simulink library "lib_HVManager_PostIMG_2017a"  (R2017a)
settings: Solver=VariableStepAuto  StartTime=0.0  StopTime=10.0  RelTol=1e-3
libraries: simulink x12, powerlib_meascontrol x3
settings Model: Creator=Vraj M  LastModifiedBy=vraj

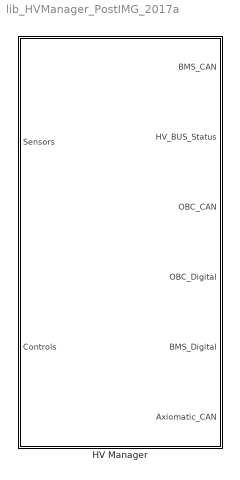
== system lib_HVManager_PostIMG_2017a ==
  HV Manager : Subsystem

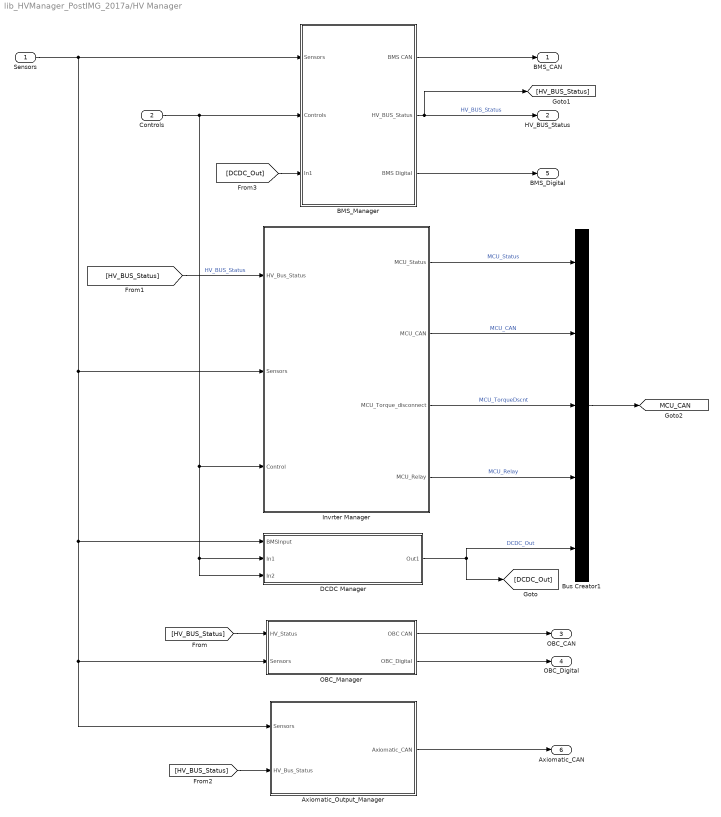
== system lib_HVManager_PostIMG_2017a/HV Manager ==
  Sensors : Inport
  Controls : Inport  Port=2
  Axiomatic_Output_Manager : Subsystem
  BMS_Manager : Subsystem
  Bus Creator1 : BusCreator  Inputs=5
  DCDC Manager : Subsystem
  Invrter Manager : Subsystem
  OBC_Manager : Subsystem
  BMS_CAN : Outport
  HV_BUS_Status : Outport  Port=2
  OBC_CAN : Outport  Port=3
  OBC_Digital : Outport  Port=4
  BMS_Digital : Outport  Port=5
  Axiomatic_CAN : Outport  Port=6
  tag scope: MCU_CAN=global
  wires:
  Axiomatic_Output_Manager/1(Axiomatic_CAN) -> Axiomatic_CAN/1
  BMS_Manager/3(BMS Digital) -> BMS_Digital/1
  BMS_Manager/1(BMS CAN) -> BMS_CAN/1
  Controls/1 -> Invrter Manager/3(Control), DCDC Manager/3(In2), DCDC Manager/2(In1), BMS_Manager/2(Controls)
  OBC_Manager/2(OBC_Digital) -> OBC_Digital/1
  OBC_Manager/1(OBC CAN) -> OBC_CAN/1
  [HV_BUS_Status] -> OBC_Manager/1(HV_Status)
  BMS_Manager/2(HV_BUS_Status) -> HV_BUS_Status/1, [HV_BUS_Status]  "HV_BUS_Status"
  [HV_BUS_Status] -> Axiomatic_Output_Manager/2(HV_Bus_Status)
  [HV_BUS_Status] -> Invrter Manager/1(HV_Bus_Status)  "HV_BUS_Status"
  Sensors/1 -> OBC_Manager/2(Sensors), Axiomatic_Output_Manager/1(Sensors), DCDC Manager/1(BMSInput), Invrter Manager/2(Sensors), BMS_Manager/1(Sensors)
  Invrter Manager/1(MCU_Status) -> Bus Creator1/1  "MCU_Status"
  Invrter Manager/2(MCU_CAN) -> Bus Creator1/2  "MCU_CAN"
  Invrter Manager/3(MCU_Torque_disconnect) -> Bus Creator1/3  "MCU_TorqueDscnt"
  Invrter Manager/4(MCU_Relay) -> Bus Creator1/4  "MCU_Relay"
  Bus Creator1/1 -> [MCU_CAN]
  DCDC Manager/1(Out1) -> Bus Creator1/5, [DCDC_Out]  "DCDC_Out"
  [DCDC_Out] -> BMS_Manager/3(In1)

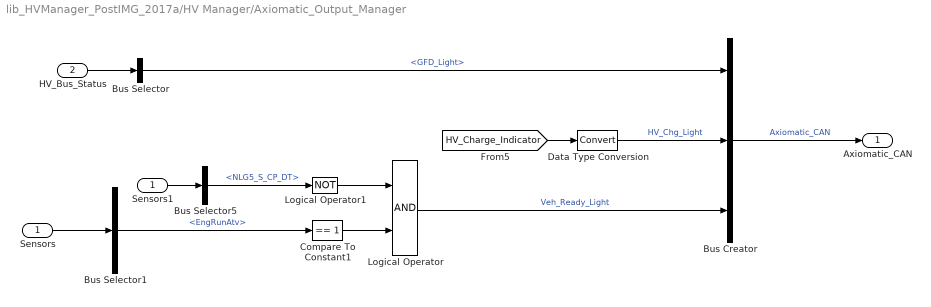
== system lib_HVManager_PostIMG_2017a/HV Manager/Axiomatic_Output_Manager ==
  Sensors : Inport
  HV_Bus_Status : Inport  Port=2
  Bus Creator : BusCreator  Inputs=3
  Bus Selector : BusSelector  OutputSignals=GFD_Light
  Bus Selector1 : BusSelector  OutputSignals=from_CAN.fromEBCAN.from_ECM.EngRunAtv
  Bus Selector5 : BusSelector  OutputSignals=from_CAN.fromHV_CAN.from_OBC.NLG5_ST.NLG5_S_CP_DT
  Compare To Constant1 : simulink/Logic and Bit Operations/Compare To Constant  relop===  const=1  OutDataTypeStr=boolean
      link override Compare: Operator===  OutDataTypeStr=boolean
  Data Type Conversion : DataTypeConversion
  Logical Operator : Logic  AllPortsSameDT=off  OutDataTypeStr=boolean
  Logical Operator1 : Logic  Operator=NOT  AllPortsSameDT=off  OutDataTypeStr=boolean
  Sensors1 : InportShadow
  Axiomatic_CAN : Outport
  wires:
  [HV_Charge_Indicator] -> Data Type Conversion/1
  Sensors/1 -> Bus Selector1/1
  Logical Operator/1 -> Bus Creator/3  "Veh_Ready_Light"
  Data Type Conversion/1 -> Bus Creator/2  "HV_Chg_Light"
  Bus Selector/1 -> Bus Creator/1  "<GFD_Light>"
  Bus Creator/1 -> Axiomatic_CAN/1  "Axiomatic_CAN"
  HV_Bus_Status/1 -> Bus Selector/1
  Compare To Constant1/1 -> Logical Operator/2
  Logical Operator1/1 -> Logical Operator/1
  Bus Selector5/1 -> Logical Operator1/1  "<NLG5_S_CP_DT>"
  Bus Selector1/1 -> Compare To Constant1/1  "<EngRunAtv>"
  Sensors1/1 -> Bus Selector5/1

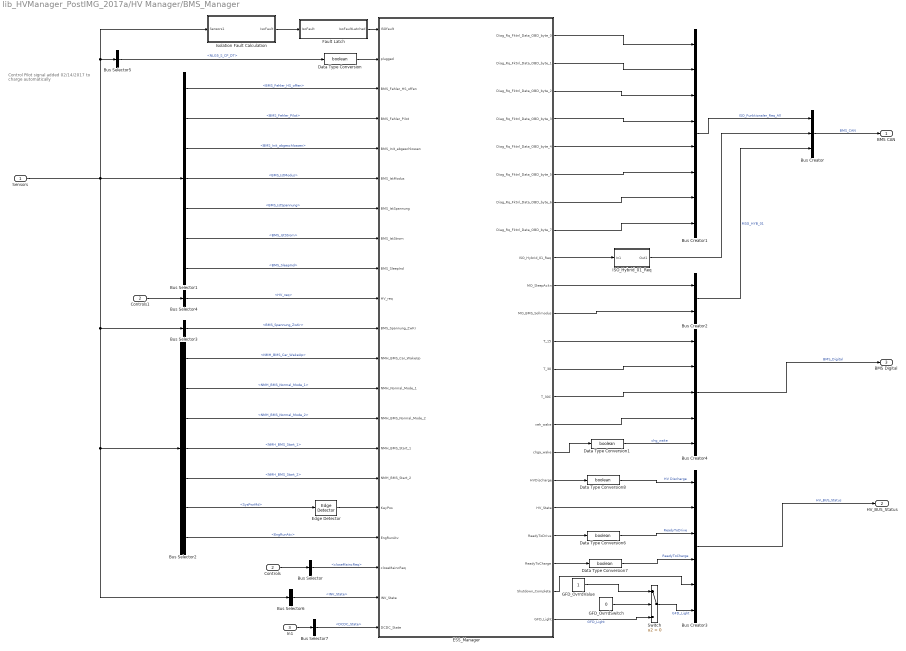
== system lib_HVManager_PostIMG_2017a/HV Manager/BMS_Manager ==
  note: Control Pilot signal added 02/14/2017
      | to charge automatically
  Sensors : Inport
  Controls : Inport  Port=2
  In1 : Inport  Port=3
  Bus Creator : BusCreator  Inputs=3
  Bus Creator1 : BusCreator  Inputs=8
  Bus Creator2 : BusCreator  Inputs=2
  Bus Creator3 : BusCreator  Inputs=6
  Bus Creator4 : BusCreator  Inputs=5
  Bus Selector : BusSelector  OutputSignals=closeMaincReq
  Bus Selector1 : BusSelector  OutputSignals=from_CAN.fromHV_CAN.from_BMSHybrid.BMS_HYB_02.BMS_Fehler_HS_offen,from_CAN.fromHV_CAN.from_BMSHybrid.BMS_HYB_02.BMS_Fehler_Pilot,from_CAN.fromHV_CAN.from_BMSHybrid.BMS_HYB_02.BMS_Init_abgeschlossen,from_CAN.fromHV_CAN.from_BMSHybrid.BMS_HYB_02.BMS_IstModus,from_CAN.fromHV_CAN.from_BMSHybrid.BMS_HYB_02.BMS_IstSpannung,from_CAN.fromHV_CAN.from_BMSHybrid.BMS_HYB_02.BMS_IstStrom,from_CAN.fromHV_CAN.from_BMSHybrid.BMS_HYB_02.BMS_SleepInd
  Bus Selector2 : BusSelector  OutputSignals=from_CAN.fromEBCAN.from_BMSAntrieb.NMH_BMS.NMH_BMS_Car_WakeUp,from_CAN.fromEBCAN.from_BMSAntrieb.NMH_BMS.NMH_BMS_Normal_Mode_1,from_CAN.fromEBCAN.from_BMSAntrieb.NMH_BMS.NMH_BMS_Normal_Mode_2,from_CAN.fromEBCAN.from_BMSAntrieb.NMH_BMS.NMH_BMS_Start_1,from_CAN.fromEBCAN.from_BMSAntrieb.NMH_BMS.NMH_BMS_Start_2,from_CAN.fromVEH_CAN.from_BCM.SysPwrMd,from_CAN.fromEBCAN.from_ECM.EngRunAtv
  Bus Selector3 : BusSelector  OutputSignals=from_CAN.fromHV_CAN.from_BMSHybrid.BMS_Spannung_ZwKr
  Bus Selector4 : BusSelector  OutputSignals=HV_req
  Bus Selector5 : BusSelector  OutputSignals=from_CAN.fromHV_CAN.from_OBC.NLG5_ST.NLG5_S_CP_DT
  Bus Selector6 : BusSelector  OutputSignals=from_CAN.fromHV_CAN.from_MCU.INV_VCU_01.INV_State
  Bus Selector7 : BusSelector  OutputSignals=DCDC_State
  Controls1 : InportShadow  Port=2
  Data Type Conversion{,1,6..8} (5 alike) : DataTypeConversion  OutDataTypeStr=boolean
  ESS_Manager : Stateflow chart  TreatAsAtomicUnit=on
  Edge Detector : powerlib_meascontrol/Logic/Edge Detector  model=Either  ic=0  Ts=0
      settings: SourceProductName=Simscape Power Systems  SourceProductBaseCode=PS
  Fault Latch : Subsystem
  GFD_OvrrdSwitch : Constant  Value=0
  GFD_OvrrdValue : Constant
  ISO_Hybrid_01_Req : Subsystem
  Isolation Fault Calculation : Subsystem
  Switch : Switch  Criteria=u2 > Threshold
  BMS CAN : Outport
  HV_BUS_Status : Outport  Port=2
  BMS Digital : Outport  Port=3
  wires:
  ISO_Hybrid_01_Req/1(Out1) -> Bus Creator/2
  ESS_Manager/9(ISO_Hybrid_01_Req) -> ISO_Hybrid_01_Req/1(In1)
  ESS_Manager/11(MO_BMS_Sollmodus) -> Bus Creator2/2
  Sensors/1 -> Bus Selector6/1, Bus Selector2/1, Bus Selector3/1, Isolation Fault Calculation/1(Sensors1), Bus Selector5/1, Bus Selector1/1
  Data Type Conversion1/1 -> Bus Creator4/5  "chg_wake"
  Bus Creator4/1 -> BMS Digital/1  "BMS_Digital"
  Bus Creator/1 -> BMS CAN/1  "BMS_CAN"
  Controls1/1 -> Bus Selector4/1
  Bus Selector/1 -> ESS_Manager/19(closeMaincReq)  "<closeMaincReq>"
  Controls/1 -> Bus Selector/1
  Bus Creator3/1 -> HV_BUS_Status/1  "HV_BUS_Status"
  ESS_Manager/18(HV_State) -> Bus Creator3/2
  ESS_Manager/15(veh_wake) -> Bus Creator4/4
  ESS_Manager/14(T_30C) -> Bus Creator4/3
  ESS_Manager/16(chga_wake) -> Data Type Conversion1/1
  ESS_Manager/13(T_30) -> Bus Creator4/2
  ESS_Manager/21(Shutdown_Complete) -> Bus Creator3/5
  ESS_Manager/20(ReadyToCharge) -> Data Type Conversion7/1
  ESS_Manager/19(ReadyToDrive) -> Data Type Conversion6/1
  ESS_Manager/17(HVDischarge) -> Data Type Conversion8/1
  Bus Creator1/1 -> Bus Creator/1  "ISO_Funktionaler_Req_All"
  Data Type Conversion8/1 -> Bus Creator3/1  "HV Discharge"
  Data Type Conversion7/1 -> Bus Creator3/4  "ReadyToCharge"
  Data Type Conversion6/1 -> Bus Creator3/3  "ReadyToDrive"
  ESS_Manager/12(T_15) -> Bus Creator4/1
  ESS_Manager/10(MO_SleepAckn) -> Bus Creator2/1
  ESS_Manager/8(Diag_Rq_Fktnl_Data_OBD_byte_7) -> Bus Creator1/8
  ESS_Manager/7(Diag_Rq_Fktnl_Data_OBD_byte_6) -> Bus Creator1/7
  ESS_Manager/6(Diag_Rq_Fktnl_Data_OBD_byte_5) -> Bus Creator1/6
  ESS_Manager/5(Diag_Rq_Fktnl_Data_OBD_byte_4) -> Bus Creator1/5
  ESS_Manager/4(Diag_Rq_Fktnl_Data_OBD_byte_3) -> Bus Creator1/4
  ESS_Manager/3(Diag_Rq_Fktnl_Data_OBD_byte_2) -> Bus Creator1/3
  ESS_Manager/2(Diag_Rq_Fktnl_Data_OBD_byte_1) -> Bus Creator1/2
  ESS_Manager/1(Diag_Rq_Fktnl_Data_OBD_byte_0) -> Bus Creator1/1
  Bus Selector5/1 -> Data Type Conversion/1  "<NLG5_S_CP_DT>"
  Bus Selector3/1 -> ESS_Manager/11(BMS_Spannung_ZwKr)  "<BMS_Spannung_ZwKr>"
  Bus Selector2/3 -> ESS_Manager/14(NMH_BMS_Normal_Mode_2)  "<NMH_BMS_Normal_Mode_2>"
  Bus Selector2/2 -> ESS_Manager/13(NMH_Normal_Mode_1)  "<NMH_BMS_Normal_Mode_1>"
  Bus Selector2/1 -> ESS_Manager/12(NMH_BMS_Car_WakeUp)  "<NMH_BMS_Car_WakeUp>"
  Bus Selector1/5 -> ESS_Manager/7(BMS_IstSpannung)  "<BMS_IstSpannung>"
  Bus Selector1/4 -> ESS_Manager/6(BMS_IstModus)  "<BMS_IstModus>"
  Bus Selector1/3 -> ESS_Manager/5(BMS_Init_abgeschlossen)  "<BMS_Init_abgeschlossen>"
  Bus Selector1/2 -> ESS_Manager/4(BMS_Fehler_Pilot)  "<BMS_Fehler_Pilot>"
  Bus Selector1/1 -> ESS_Manager/3(BMS_Fehler_HS_offen)  "<BMS_Fehler_HS_offen>"
  Switch/1 -> Bus Creator3/6  "GFD_Light"
  Isolation Fault Calculation/1(IsoFault) -> Fault Latch/1(IsoFault)
  Fault Latch/1(IsoFaultLatched) -> ESS_Manager/1(ISOfault)
  Bus Creator2/1 -> Bus Creator/3  "MSG_HYB_01"
  Bus Selector4/1 -> ESS_Manager/10(HV_req)  "<HV_req>"
  Bus Selector2/6 -> Edge Detector/1  "<SysPwrMd>"
  Edge Detector/1 -> ESS_Manager/17(KeyPos)
  Bus Selector2/7 -> ESS_Manager/18(EngRunAtv)  "<EngRunAtv>"
  Bus Selector2/5 -> ESS_Manager/16(NMH_BMS_Start_2)  "<NMH_BMS_Start_2>"
  Bus Selector2/4 -> ESS_Manager/15(NMH_BMS_Start_1)  "<NMH_BMS_Start_1>"
  Bus Selector1/7 -> ESS_Manager/9(BMS_SleepInd)  "<BMS_SleepInd>"
  Bus Selector1/6 -> ESS_Manager/8(BMS_IstStrom)  "<BMS_IstStrom>"
  Data Type Conversion/1 -> ESS_Manager/2(plugged)
  ESS_Manager/22(GFD_Light) -> Switch/3  "GFD_Light"
  GFD_OvrrdSwitch/1 -> Switch/2
  GFD_OvrrdValue/1 -> Switch/1
  Bus Selector6/1 -> ESS_Manager/20(INV_State)  "<INV_State>"
  In1/1 -> Bus Selector7/1
  Bus Selector7/1 -> ESS_Manager/21(DCDC_State)  "<DCDC_State>"

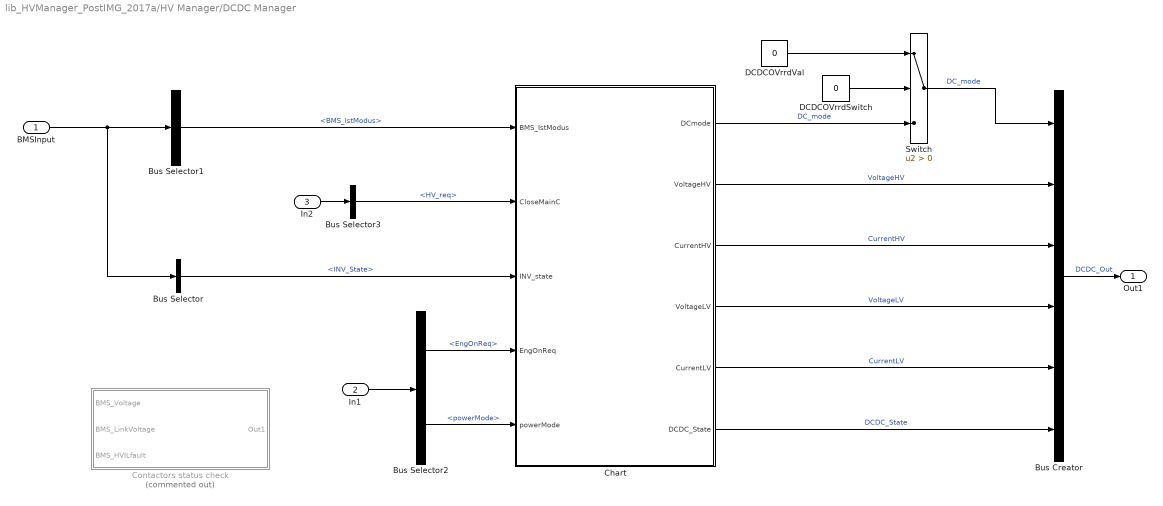
== system lib_HVManager_PostIMG_2017a/HV Manager/DCDC Manager ==
  BMSInput : Inport
  In1 : Inport  Port=2
  In2 : Inport  Port=3
  Bus Creator : BusCreator  Inputs=6
  Bus Selector : BusSelector  OutputSignals=from_CAN.fromHV_CAN.from_MCU.INV_VCU_01.INV_State
  Bus Selector1 : BusSelector  OutputSignals=from_CAN.fromHV_CAN.from_BMSHybrid.BMS_HYB_02.BMS_IstModus
  Bus Selector2 : BusSelector  OutputSignals=EngOnReq,powerMode
  Bus Selector3 : BusSelector  OutputSignals=HV_req
  Chart : Stateflow chart  RequirementInfo={} %GIDa_d26a8659_2f91_4e0f_9a85_a466cd76580c  TreatAsAtomicUnit=on
  Contactors status check : Subsystem  Commented=on
  DCDCOVrrdSwitch : Constant  Value=0
  DCDCOVrrdVal : Constant  Value=0
  Switch : Switch  Criteria=u2 > Threshold
  Out1 : Outport
  wires:
  BMSInput/1 -> Bus Selector/1, Bus Selector1/1
  Bus Selector/1 -> Chart/3(INV_state)  "<INV_State>"
  Switch/1 -> Bus Creator/1  "DC_mode"
  Chart/5(CurrentLV) -> Bus Creator/5  "CurrentLV"
  Chart/4(VoltageLV) -> Bus Creator/4  "VoltageLV"
  Chart/3(CurrentHV) -> Bus Creator/3  "CurrentHV"
  Chart/2(VoltageHV) -> Bus Creator/2  "VoltageHV"
  Bus Creator/1 -> Out1/1  "DCDC_Out"
  Chart/6(DCDC_State) -> Bus Creator/6  "DCDC_State"
  Chart/1(DCmode) -> Switch/3  "DC_mode"
  DCDCOVrrdSwitch/1 -> Switch/2
  DCDCOVrrdVal/1 -> Switch/1
  In1/1 -> Bus Selector2/1
  Bus Selector2/2 -> Chart/5(powerMode)  "<powerMode>"
  Bus Selector1/1 -> Chart/1(BMS_IstModus)  "<BMS_IstModus>"
  Bus Selector2/1 -> Chart/4(EngOnReq)  "<EngOnReq>"
  In2/1 -> Bus Selector3/1
  Bus Selector3/1 -> Chart/2(CloseMainC)  "<HV_req>"

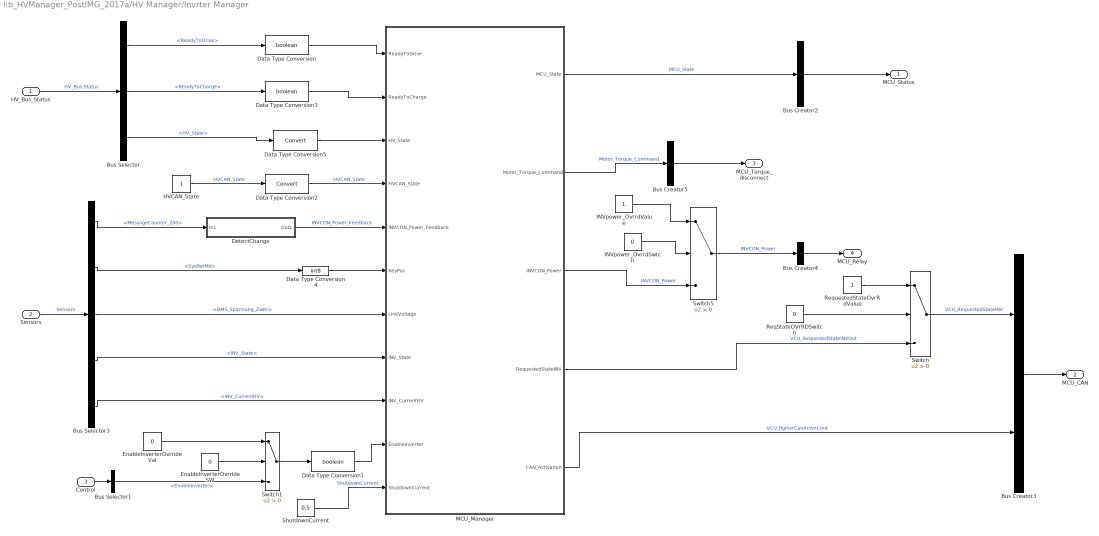
== system lib_HVManager_PostIMG_2017a/HV Manager/Invrter Manager ==
  HV_Bus_Status : Inport
  Sensors : Inport  Port=2
  Control : Inport  Port=3
  Bus Creator2 : BusCreator  Inputs=1
  Bus Creator3 : BusCreator  Inputs=2
  Bus Creator4 : BusCreator  Inputs=1
  Bus Creator5 : BusCreator  Inputs=1
  Bus Selector : BusSelector  OutputSignals=ReadyToDrive,ReadyToCharge,HV_State
  Bus Selector1 : BusSelector  OutputSignals=EnableInverter
  Bus Selector3 : BusSelector  OutputSignals=from_CAN.fromHV_CAN.from_MCU.INV_VCU_01.MessageCounter_200,from_CAN.fromVEH_CAN.from_BCM.SysPwrMd,from_CAN.fromHV_CAN.from_BMSHybrid.BMS_Spannung_ZwKr,from_CAN.fromHV_CAN.from_MCU.INV_VCU_01.INV_State,from_CAN.fromHV_CAN.from_MCU.INV_VCU_01.INV_CurrentHV
  Data Type Conversion : DataTypeConversion  OutDataTypeStr=boolean
  Data Type Conversion1 : DataTypeConversion  OutDataTypeStr=boolean
  Data Type Conversion2 : DataTypeConversion
  Data Type Conversion3 : DataTypeConversion  OutDataTypeStr=boolean
  Data Type Conversion4 : DataTypeConversion  OutDataTypeStr=int8
  Data Type Conversion5 : DataTypeConversion
  DetectChange : Subsystem
  EnableInverterOvrrideSW : Constant  Value=0
  EnableInverterOvrrideVal : Constant  Value=0
  HVCAN_State : Constant
  INVpower_OvrrdSwtch : Constant  Value=0
  INVpower_OvrrdValue : Constant
  "MCU_Manager " : Stateflow chart  RequirementInfo={} %GIDa_847f7ea3_a24c_4f3c_837a_ca9eed8e7071  TreatAsAtomicUnit=on
  ReqStateOVrRDSwitch : Constant  Value=0
  RequestedStateOvrRdValue : Constant
  ShutdownCurrent : Constant  Value=0.5
  Switch : Switch  Criteria=u2 > Threshold
  Switch1 : Switch  Criteria=u2 > Threshold
  Switch5 : Switch  Criteria=u2 > Threshold
  MCU_Status : Outport
  MCU_CAN : Outport  Port=2
  MCU_Torque_disconnect : Outport  Port=3
  MCU_Relay : Outport  Port=4
  wires:
  HVCAN_State/1 -> Data Type Conversion2/1  "HVCAN_State"
  Bus Selector3/4 -> "MCU_Manager "/8(INV_State)  "<INV_State>"
  Data Type Conversion1/1 -> "MCU_Manager "/10(EnableInverter)
  Data Type Conversion/1 -> "MCU_Manager "/1(ReadyToDrive)
  Bus Creator5/1 -> MCU_Torque_disconnect/1
  "MCU_Manager "/2(Motor_Torque_Command) -> Bus Creator5/1  "Motor_Torque_Command"
  Bus Creator4/1 -> MCU_Relay/1
  Switch5/1 -> Bus Creator4/1  "INVCON_Power"
  Bus Creator2/1 -> MCU_Status/1
  "MCU_Manager "/1(MCU_State) -> Bus Creator2/1  "MCU_State"
  Bus Selector3/5 -> "MCU_Manager "/9(INV_CurrentHV)  "<INV_CurrentHV>"
  ShutdownCurrent/1 -> "MCU_Manager "/11(ShutdownCurrent)  "ShutdownCurrent"
  Bus Selector/1 -> Data Type Conversion/1  "<ReadyToDrive>"
  HV_Bus_Status/1 -> Bus Selector/1  "HV_Bus Status"
  EnableInverterOvrrideVal/1 -> Switch1/1
  Sensors/1 -> Bus Selector3/1  "Sensors"
  Bus Creator3/1 -> MCU_CAN/1
  Data Type Conversion2/1 -> "MCU_Manager "/4(HVCAN_State)  "HVCAN_State"
  Bus Selector/2 -> Data Type Conversion3/1  "<ReadyToCharge>"
  Data Type Conversion3/1 -> "MCU_Manager "/2(ReadyToCharge)
  DetectChange/1(Out1) -> "MCU_Manager "/5(INVCON_Power_Feedback)  "INVCON_Power_Feedback"
  "MCU_Manager "/5(CAN_Activation) -> Bus Creator3/2  "VCU_flgInvrCanActvnCmd"
  Switch/1 -> Bus Creator3/1  "VCU_RequestedStateINV"
  "MCU_Manager "/4(RequestedStateINV) -> Switch/3  "VCU_RequestedStateINVOut"
  ReqStateOVrRDSwitch/1 -> Switch/2
  RequestedStateOvrRdValue/1 -> Switch/1
  Control/1 -> Bus Selector1/1
  Switch1/1 -> Data Type Conversion1/1
  Bus Selector1/1 -> Switch1/3  "<EnableInverter>"
  EnableInverterOvrrideSW/1 -> Switch1/2
  Bus Selector3/3 -> "MCU_Manager "/7(LinkVoltage)  "<BMS_Spannung_ZwKr>"
  Bus Selector3/2 -> Data Type Conversion4/1  "<SysPwrMd>"
  Data Type Conversion4/1 -> "MCU_Manager "/6(KeyPos)
  Bus Selector3/1 -> DetectChange/1(In1)  "<MessageCounter_200>"
  Bus Selector/3 -> Data Type Conversion5/1  "<HV_State>"
  Data Type Conversion5/1 -> "MCU_Manager "/3(HV_State)
  INVpower_OvrrdSwtch/1 -> Switch5/2
  INVpower_OvrrdValue/1 -> Switch5/1
  "MCU_Manager "/3(INVCON_Power) -> Switch5/3  "INVCON_Power"

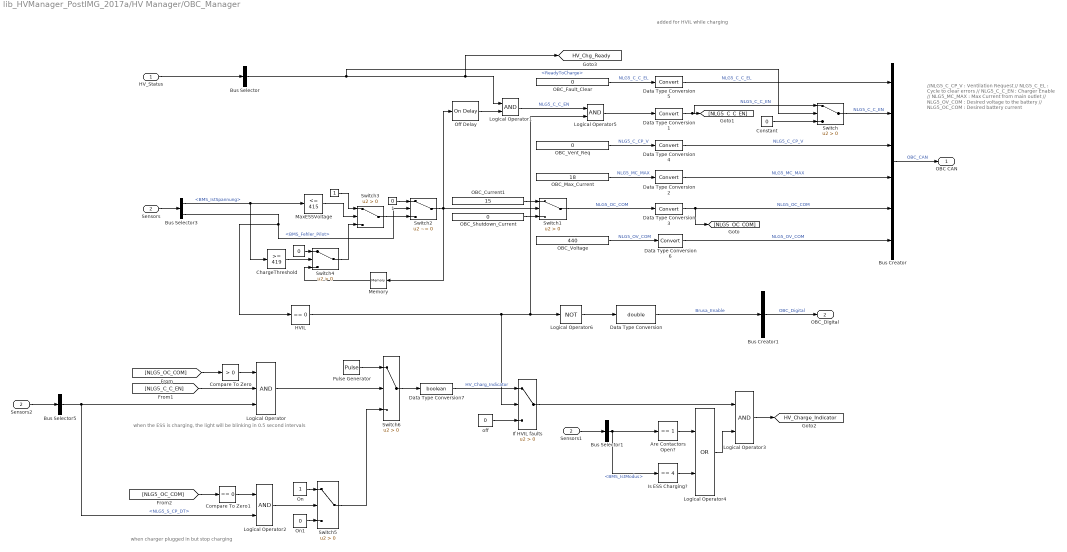
== system lib_HVManager_PostIMG_2017a/HV Manager/OBC_Manager ==
  note: added for HVIL
      | while charging
  note: //NLG5_C_CP_V : Ventilation Request
      | // NLG5_C_EL : Cycle to clear errors
      | // NLG5_C_C_EN : Charger Enable
      | // NLG5_MC_MAX : Max Current from main outlet
      | // NLG5_OV_COM : Desired voltage to the battery
      | // NLG5_OC_COM : Desired battery current
  note: when charger plugged in but stop charging
  note: when the ESS is charging, the light will be blinking in 0.5 second intervals
  HV_Status : Inport
  Sensors : Inport  Port=2
  " " : Constant
  "   " : Constant  Value=0
  "   1" : Constant  Value=0
  Are Contactors Open? : simulink/Logic and Bit Operations/Compare To Constant  relop===  const=1  OutDataTypeStr=boolean
      link override Compare: Operator===  OutDataTypeStr=boolean
  Bus Creator : BusCreator  Inputs=6
  Bus Creator1 : BusCreator  Inputs=1
  Bus Selector : BusSelector  OutputSignals=ReadyToCharge
  Bus Selector1 : BusSelector  OutputSignals=from_CAN.fromHV_CAN.from_BMSHybrid.BMS_HYB_02.BMS_IstModus
  Bus Selector3 : BusSelector  OutputSignals=from_CAN.fromHV_CAN.from_BMSHybrid.BMS_HYB_02.BMS_IstSpannung,from_CAN.fromHV_CAN.from_BMSHybrid.BMS_HYB_02.BMS_Fehler_Pilot
  Bus Selector5 : BusSelector  OutputSignals=from_CAN.fromHV_CAN.from_OBC.NLG5_ST.NLG5_S_CP_DT
  ChargeThreshold : simulink/Logic and Bit Operations/Compare To Constant  relop=>=  const=419  OutDataTypeStr=boolean
      link override Compare: Operator=>=  OutDataTypeStr=boolean
  Compare To Zero : simulink/Logic and Bit Operations/Compare To Zero  relop=>  OutDataTypeStr=boolean
      link override Compare: Operator=>  OutDataTypeStr=boolean
  Compare To Zero1 : simulink/Logic and Bit Operations/Compare To Zero  relop===  OutDataTypeStr=boolean
      link override Compare: Operator===  OutDataTypeStr=boolean
  Constant : Constant  Value=0
  Data Type Conversion : DataTypeConversion  OutDataTypeStr=double
  Data Type Conversion{1..6} (6 alike) : DataTypeConversion
  Data Type Conversion7 : DataTypeConversion  OutDataTypeStr=boolean
  HVIL : simulink/Logic and Bit Operations/Compare To Constant  relop===  const=0  OutDataTypeStr=boolean
      link override Compare: Operator===  OutDataTypeStr=boolean
  If HVIL faults : Switch  Criteria=u2 > Threshold
  Is ESS Charging? : simulink/Logic and Bit Operations/Compare To Constant  relop===  const=4  OutDataTypeStr=boolean
      link override Compare: Operator===  OutDataTypeStr=boolean
  Logical Operator : Logic  Inputs=3  AllPortsSameDT=off  OutDataTypeStr=boolean
  Logical Operator{1..3,5} (4 alike) : Logic  AllPortsSameDT=off  OutDataTypeStr=boolean
  Logical Operator4 : Logic  Operator=OR  AllPortsSameDT=off  OutDataTypeStr=boolean
  Logical Operator6 : Logic  Operator=NOT  Inputs=3  AllPortsSameDT=off  OutDataTypeStr=boolean
  MaxESSVoltage : simulink/Logic and Bit Operations/Compare To Constant  relop=<=  const=415  OutDataTypeStr=boolean
      link override Compare: Operator=<=  OutDataTypeStr=boolean
  Memory : Memory  InheritSampleTime=on
  OBC_Current1 : Constant  Value=15
  OBC_Fault_Clear : Constant  Value=0
  OBC_Max_Current : Constant  Value=18
  OBC_Shutdown_Current : Constant  Value=0
  OBC_Vent_Req : Constant  Value=0
  OBC_Voltage : Constant  Value=440
  Off Delay : powerlib_meascontrol/Logic/On Delay  DelayType=Off delay  delay=30  ic=0  Ts=0
      settings: SourceProductName=Simscape Power Systems
  On : Constant
  On1 : Constant  Value=0
  Pulse Generator : DiscretePulseGenerator  PulseType=Time based  Period=1  PulseWidth=50
  Sensors1 : InportShadow  Port=2
  Sensors2 : InportShadow  Port=2
  Switch{,1,3..6} (6 alike) : Switch  Criteria=u2 > Threshold
  Switch2 : Switch  Criteria=u2 ~= 0
  off : Constant  Value=0
  OBC CAN : Outport
  OBC_Digital : Outport  Port=2
  tag scope: HV_Charge_Indicator=global, HV_Chg_Ready=global
  wires:
  Data Type Conversion7/1 -> If HVIL faults/1  "HV_Charg_Indicator"
  OBC_Voltage/1 -> Data Type Conversion6/1  "NLG5_OV_COM"
  OBC_Max_Current/1 -> Data Type Conversion2/1  "NLG5_MC_MAX"
  OBC_Fault_Clear/1 -> Data Type Conversion5/1  "NLG5_C_C_EL"
  OBC_Vent_Req/1 -> Data Type Conversion4/1  "NLG5_C_CP_V"
  Switch1/1 -> Data Type Conversion3/1  "NLG5_OC_COM"
  Logical Operator1/1 -> Logical Operator5/1  "NLG5_C_C_EN"
  Data Type Conversion1/1 -> Switch/1, [NLG5_C_C_EN]  "NLG5_C_C_EN"
  Switch4/1 -> Switch3/3
  Memory/1 -> Switch4/3
  OBC_Shutdown_Current/1 -> Switch1/3
  " "/1 -> Switch3/1
  ChargeThreshold/1 -> Switch4/2
  "   "/1 -> Switch4/1
  Switch2/1 -> Memory/1, Off Delay/1, Switch1/2
  OBC_Current1/1 -> Switch1/1
  Data Type Conversion3/1 -> Bus Creator/5, [NLG5_OC_COM]  "NLG5_OC_COM"
  Data Type Conversion6/1 -> Bus Creator/6  "NLG5_OV_COM"
  Data Type Conversion4/1 -> Bus Creator/3  "NLG5_C_CP_V"
  Data Type Conversion5/1 -> Bus Creator/1  "NLG5_C_C_EL"
  Data Type Conversion2/1 -> Bus Creator/4  "NLG5_MC_MAX"
  Bus Selector3/1 -> ChargeThreshold/1, MaxESSVoltage/1  "<BMS_IstSpannung>"
  Off Delay/1 -> Logical Operator1/2
  Bus Selector/1 -> Switch/2, Logical Operator1/1, [HV_Chg_Ready]  "<ReadyToCharge>"
  MaxESSVoltage/1 -> Switch3/2
  HV_Status/1 -> Bus Selector/1
  Bus Creator/1 -> OBC CAN/1  "OBC_CAN"
  Sensors/1 -> Bus Selector3/1
  [NLG5_OC_COM] -> Compare To Zero/1
  Compare To Zero/1 -> Logical Operator/1
  [NLG5_C_C_EN] -> Logical Operator/2
  Logical Operator/1 -> Switch6/2
  Pulse Generator/1 -> Switch6/1
  [NLG5_OC_COM] -> Compare To Zero1/1
  Compare To Zero1/1 -> Logical Operator2/1
  Logical Operator2/1 -> Switch5/2
  On/1 -> Switch5/1
  On1/1 -> Switch5/3
  Switch5/1 -> Switch6/3
  Switch6/1 -> Data Type Conversion7/1
  Bus Selector3/2 -> HVIL/1, Switch2/2  "<BMS_Fehler_Pilot>"
  Data Type Conversion/1 -> Bus Creator1/1  "Brusa_Enable"
  Bus Creator1/1 -> OBC_Digital/1  "OBC_Digital"
  Switch3/1 -> Switch2/3
  "   1"/1 -> Switch2/1
  HVIL/1 -> Logical Operator5/2, Logical Operator6/1, If HVIL faults/2
  If HVIL faults/1 -> Logical Operator3/1
  off/1 -> If HVIL faults/3
  Logical Operator3/1 -> [HV_Charge_Indicator]
  Sensors1/1 -> Bus Selector1/1
  Are Contactors Open?/1 -> Logical Operator4/1
  Bus Selector1/1 -> Is ESS Charging?/1, Are Contactors Open?/1  "<BMS_IstModus>"
  Is ESS Charging?/1 -> Logical Operator4/2
  Logical Operator4/1 -> Logical Operator3/2
  Logical Operator5/1 -> Data Type Conversion1/1
  Logical Operator6/1 -> Data Type Conversion/1
  Constant/1 -> Switch/3
  Switch/1 -> Bus Creator/2  "NLG5_C_C_EN"
  Bus Selector5/1 -> Logical Operator2/2, Logical Operator/3  "<NLG5_S_CP_DT>"
  Sensors2/1 -> Bus Selector5/1

== system lib_HVManager_PostIMG_2017a/HV Manager/BMS_Manager/Fault Latch ==
  IsoFault : Inport
  Off Delay : powerlib_meascontrol/Logic/On Delay  DelayType=Off delay  delay=3  ic=0  Ts=0
      settings: SourceProductName=Simscape Power Systems
  IsoFaultLatched : Outport
  wires:
  IsoFault/1 -> Off Delay/1
  Off Delay/1 -> IsoFaultLatched/1

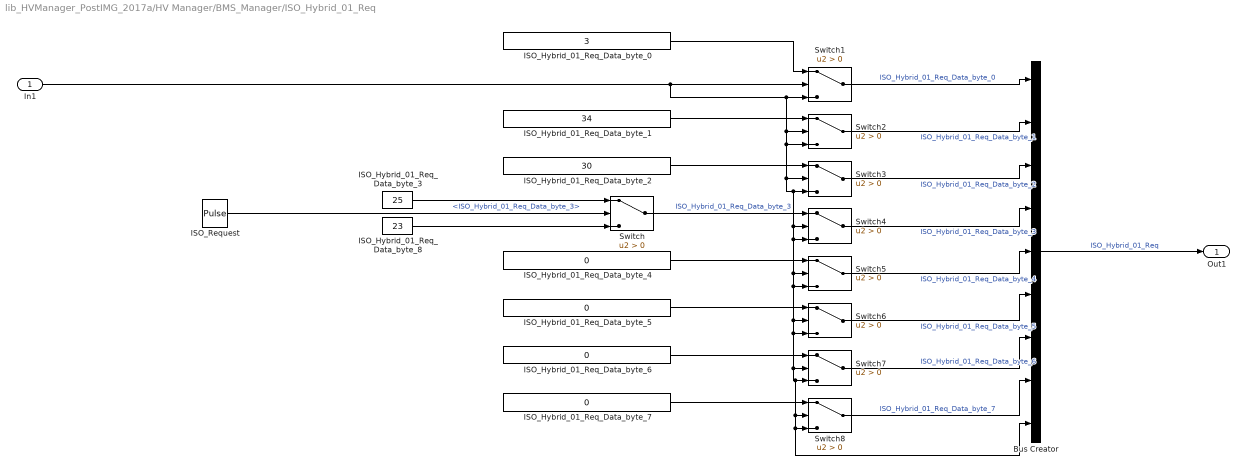
== system lib_HVManager_PostIMG_2017a/HV Manager/BMS_Manager/ISO_Hybrid_01_Req ==
  In1 : Inport
  Bus Creator : BusCreator  Inputs=9
  ISO_Hybrid_01_Req_Data_byte_0 : Constant  Value=3
  ISO_Hybrid_01_Req_Data_byte_1 : Constant  Value=34
  ISO_Hybrid_01_Req_Data_byte_2 : Constant  Value=30
  ISO_Hybrid_01_Req_Data_byte_3 : Constant  Value=25
  ISO_Hybrid_01_Req_Data_byte_{4..7} (4 alike) : Constant  Value=0
  ISO_Hybrid_01_Req_Data_byte_8 : Constant  Value=23
  ISO_Request : DiscretePulseGenerator  PulseType=Time based  Period=0.5  PulseWidth=50  SampleTime=-1
  Switch{,1..8} (9 alike) : Switch  Criteria=u2 > Threshold
  Out1 : Outport
  wires:
  Bus Creator/1 -> Out1/1  "ISO_Hybrid_01_Req"
  Switch6/1 -> Bus Creator/6  "ISO_Hybrid_01_Req_Data_byte_5"
  ISO_Hybrid_01_Req_Data_byte_8/1 -> Switch/3
  Switch5/1 -> Bus Creator/5  "ISO_Hybrid_01_Req_Data_byte_4"
  Switch3/1 -> Bus Creator/3  "ISO_Hybrid_01_Req_Data_byte_2"
  ISO_Hybrid_01_Req_Data_byte_3/1 -> Switch/1
  Switch1/1 -> Bus Creator/1  "ISO_Hybrid_01_Req_Data_byte_0"
  Switch7/1 -> Bus Creator/7  "ISO_Hybrid_01_Req_Data_byte_6"
  Switch2/1 -> Bus Creator/2  "ISO_Hybrid_01_Req_Data_byte_1"
  Switch8/1 -> Bus Creator/8  "ISO_Hybrid_01_Req_Data_byte_7"
  Switch4/1 -> Bus Creator/4  "ISO_Hybrid_01_Req_Data_byte_3"
  ISO_Hybrid_01_Req_Data_byte_0/1 -> Switch1/1
  In1/1 -> Switch2/2, Switch3/3, Switch4/3, Switch5/3, Switch6/3, Switch7/2, Switch7/3, Switch8/2, Bus Creator/9, Switch8/3, Switch6/2, Switch5/2, Switch4/2, Switch3/2, Switch2/3, Switch1/3, Switch1/2
  ISO_Hybrid_01_Req_Data_byte_1/1 -> Switch2/1
  ISO_Hybrid_01_Req_Data_byte_2/1 -> Switch3/1
  Switch/1 -> Switch4/1  "ISO_Hybrid_01_Req_Data_byte_3"
  ISO_Hybrid_01_Req_Data_byte_4/1 -> Switch5/1
  ISO_Hybrid_01_Req_Data_byte_5/1 -> Switch6/1
  ISO_Hybrid_01_Req_Data_byte_6/1 -> Switch7/1
  ISO_Hybrid_01_Req_Data_byte_7/1 -> Switch8/1
  ISO_Request/1 -> Switch/2  "<ISO_Hybrid_01_Req_Data_byte_3>"

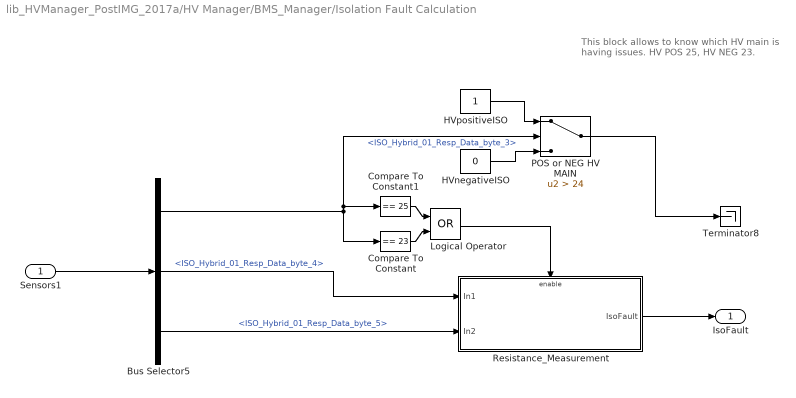
== system lib_HVManager_PostIMG_2017a/HV Manager/BMS_Manager/Isolation Fault Calculation ==
  note: This block  allows to know which HV main
      | is having issues. HV POS 25, HV NEG 23.
  Sensors1 : Inport
  Bus Selector5 : BusSelector  OutputSignals=from_CAN.fromEBCAN.from_BMSAntrieb.ISO_Hybrid_01_Resp_Data.ISO_Hybrid_01_Resp_Data_byte_3,from_CAN.fromEBCAN.from_BMSAntrieb.ISO_Hybrid_01_Resp_Data.ISO_Hybrid_01_Resp_Data_byte_4,from_CAN.fromEBCAN.from_BMSAntrieb.ISO_Hybrid_01_Resp_Data.ISO_Hybrid_01_Resp_Data_byte_5
  Compare To Constant : simulink/Logic and Bit Operations/Compare To Constant  relop===  const=23  OutDataTypeStr=boolean
      link override Compare: Operator===  OutDataTypeStr=boolean
  Compare To Constant1 : simulink/Logic and Bit Operations/Compare To Constant  relop===  const=25  OutDataTypeStr=boolean
      link override Compare: Operator===  OutDataTypeStr=boolean
  HVnegativeISO : Constant  Value=0
  HVpositiveISO : Constant
  Logical Operator : Logic  Operator=OR  AllPortsSameDT=off  OutDataTypeStr=boolean
  POS or NEG HV MAIN : Switch  Criteria=u2 > Threshold  Threshold=24
  Resistance_Measurement : Subsystem
  Terminator8 : Terminator
  IsoFault : Outport
  wires:
  Resistance_Measurement/1(IsoFault) -> IsoFault/1
  POS or NEG HV MAIN/1 -> Terminator8/1
  Bus Selector5/2 -> Resistance_Measurement/1(In1)  "<ISO_Hybrid_01_Resp_Data_byte_4>"
  Bus Selector5/3 -> Resistance_Measurement/2(In2)  "<ISO_Hybrid_01_Resp_Data_byte_5>"
  Sensors1/1 -> Bus Selector5/1
  HVpositiveISO/1 -> POS or NEG HV MAIN/1
  Bus Selector5/1 -> POS or NEG HV MAIN/2, Compare To Constant1/1, Compare To Constant/1  "<ISO_Hybrid_01_Resp_Data_byte_3>"
  HVnegativeISO/1 -> POS or NEG HV MAIN/3
  Compare To Constant1/1 -> Logical Operator/1
  Compare To Constant/1 -> Logical Operator/2
  Logical Operator/1 -> Resistance_Measurement/Enable

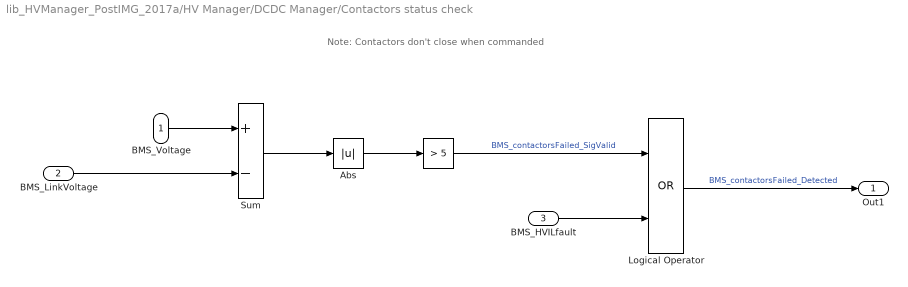
== system lib_HVManager_PostIMG_2017a/HV Manager/DCDC Manager/Contactors status check ==
  note: Note: Contactors don't close when commanded
  BMS_Voltage : Inport
  BMS_LinkVoltage : Inport  Port=2
  BMS_HVILfault : Inport  Port=3
  " " : simulink/Logic and Bit Operations/Compare To Constant  relop=>  const=5  OutDataTypeStr=boolean
      link override Compare: Operator=>  OutDataTypeStr=boolean
  Abs : Abs
  Logical Operator : Logic  Operator=OR  AllPortsSameDT=off  OutDataTypeStr=boolean
  Sum : Sum  Inputs=+-
  Out1 : Outport
  wires:
  BMS_Voltage/1 -> Sum/1
  Logical Operator/1 -> Out1/1  "BMS_contactorsFailed_Detected"
  Sum/1 -> Abs/1
  Abs/1 -> " "/1
  BMS_LinkVoltage/1 -> Sum/2
  BMS_HVILfault/1 -> Logical Operator/2
  " "/1 -> Logical Operator/1  "BMS_contactorsFailed_SigValid"

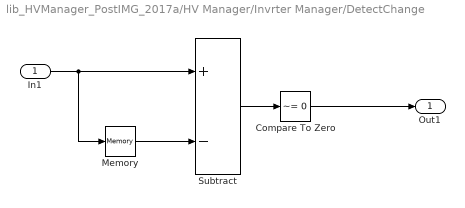
== system lib_HVManager_PostIMG_2017a/HV Manager/Invrter Manager/DetectChange ==
  In1 : Inport
  Compare To Zero : simulink/Logic and Bit Operations/Compare To Zero  relop=~=  OutDataTypeStr=boolean
  Memory : Memory
  Subtract : Sum  Inputs=+-
  Out1 : Outport
  wires:
  Memory/1 -> Subtract/2
  Compare To Zero/1 -> Out1/1
  Subtract/1 -> Compare To Zero/1
  In1/1 -> Subtract/1, Memory/1

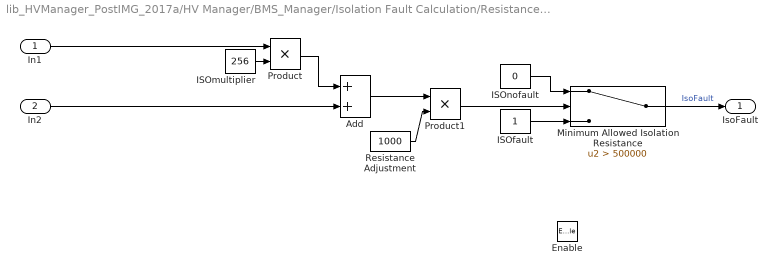
== system lib_HVManager_PostIMG_2017a/HV Manager/BMS_Manager/Isolation Fault Calculation/Resistance_Measurement ==
  In1 : Inport
  In2 : Inport  Port=2
  Enable : EnablePort
  Add : Sum
  ISOfault : Constant
  ISOmultiplier : Constant  Value=256
  ISOnofault : Constant  Value=0
  Minimum Allowed Isolation Resistance : Switch  Criteria=u2 > Threshold  Threshold=500000
  Product : Product
  Product1 : Product
  Resistance Adjustment : Constant  Value=1000
  IsoFault : Outport
  wires:
  Minimum Allowed Isolation Resistance/1 -> IsoFault/1  "IsoFault"
  ISOnofault/1 -> Minimum Allowed Isolation Resistance/1
  Resistance Adjustment/1 -> Product1/2
  Product1/1 -> Minimum Allowed Isolation Resistance/2
  ISOfault/1 -> Minimum Allowed Isolation Resistance/3
  Add/1 -> Product1/1
  Product/1 -> Add/1
  In2/1 -> Add/2
  In1/1 -> Product/1
  ISOmultiplier/1 -> Product/2

== stateflow chart lib_HVManager_PostIMG_2017a/HV Manager/DCDC Manager/Chart ==
  state Power_On
    entry: DCmode = 1;
    DCDC_State = 4;
    VoltageHV = 0;
    VoltageLV =14;
    CurrentHV = 15;
    CurrentLV = 173;
  state Delay1
    entry: DCDC_State = 3
  state Delay
    entry: DCDC_State = 2
  state DCDC_Off
    entry: DCDC_State = 1;
    DCmode = 0;
  Delay1 -> Power_On : after(3,sec)
  Power_On -> DCDC_Off : [CloseMainC == 0 || EngOnReq == 1]
  Delay -> Delay1 : [BMS_IstModus>=1&&BMS_IstModus<5]
  DCDC_Off -> Delay : [(INV_state == 3 || INV_state == 8) && (powerMode ==1|| powerMode == 2 || powerMode == 3)]
  (default) -> DCDC_Off
  data: BMS_IstModus input; CloseMainC input; DCmode output; VoltageHV output; CurrentHV output; VoltageLV output; CurrentLV output; INV_state input; DCDC_State output; EngOnReq input; powerMode input

== stateflow chart lib_HVManager_PostIMG_2017a/HV Manager/BMS_Manager/ESS_Manager ==
  state Ground_Fault
    entry:
    HV_State=-7;
    GFD_Light=1
  state Fault_light_OFF
    entry: GFD_Light=0;
  state Voltage_Fault
  state HVIL_Fault
    entry: MO_BMS_Sollmodus=0;
    HV_State=-8
  state HV_Startup
    state BMS_Wake
      entry:  HV_State=1;
      T_15=1;
      HVDischarge=0;
    state Clear_Faults
      entry:
      Diag_Rq_Fktnl_Data_OBD_byte_0 =1;
      Diag_Rq_Fktnl_Data_OBD_byte_1=4;
      Diag_Rq_Fktnl_Data_OBD_byte_2=0;
      Diag_Rq_Fktnl_Data_OBD_byte_3=0;
      Diag_Rq_Fktnl_Data_OBD_byte_4=0;
      Diag_Rq_Fktnl_Data_OBD_byte_5=0;
      Diag_Rq_Fktnl_Data_OBD_byte_6=0;
      Diag_Rq_Fktnl_Data_OBD_byte_7=0;
      HV_State=2;
    state Charge_Wake
      entry: chga_wake=1;
      HV_State=3;
    state Drive_Wake
      entry: veh_wake=1;
      HV_State=8;
    state BMS_Enable_Charge
      entry: MO_BMS_Sollmodus=0;
      HV_State=4;
    state BMS_Enable_Drive
      entry: MO_BMS_Sollmodus=0;
      HV_State=9;
    state Power_Contactors_Drive
      en:
      MO_BMS_Sollmodus=0;
      T_30C=1;
      HV_State=10;
    state Power_Contactors_Charge
      en: MO_BMS_Sollmodus=0;
      T_30C=1;
      HV_State=5;
    state Close_Contactors_Drive
      entry:
      MO_BMS_Sollmodus=1;
      HV_State=11;
    state Close_Contactors_Charge
      entry:
      MO_BMS_Sollmodus=1;
      HV_State=6;
    state Time_delay
    state Ready_to_Charge
      entry: ReadyToCharge=1;
      ISO_Hybrid_01_Req = 1;
      HV_State=7;
    state Ready_to_Drive
      entry: ReadyToDrive=1;
      ISO_Hybrid_01_Req = 1;
      HV_State=12;
    (default) -> BMS_Wake
    BMS_Wake -> Clear_Faults : after(0.1,sec)
    Clear_Faults -> Charge_Wake [order 1] : [plugged]
    Clear_Faults -> Drive_Wake [order 2] : after(0.15,sec)
    Drive_Wake -> BMS_Enable_Drive : [BMS_Fehler_Pilot==0 ]
    Charge_Wake -> BMS_Enable_Charge : [BMS_Fehler_Pilot==0 ]
    BMS_Enable_Charge -> Power_Contactors_Charge : [BMS_Init_abgeschlossen]
    BMS_Enable_Drive -> Power_Contactors_Drive : [BMS_Init_abgeschlossen]
    Power_Contactors_Drive -> Close_Contactors_Drive : [closeMaincReq]
    Power_Contactors_Charge -> Close_Contactors_Charge : [closeMaincReq]
    Close_Contactors_Charge -> Time_delay : [BMS_Fehler_HS_offen==0&&(BMS_IstModus==4||BMS_IstModus==1)]
    Close_Contactors_Drive -> Ready_to_Drive : [BMS_Fehler_HS_offen==0&&BMS_IstModus==1]
    Time_delay -> Ready_to_Charge : after(1,sec)
    Ready_to_Drive -> Ready_to_Charge : [plugged]
    Ready_to_Charge -> Ready_to_Drive : [plugged==0]
  note: // Rev 2_14_2017
      | Added plugged to Off-On transition
      | Added EnableInverter to charge path
      | Changed IstModus to 1 at the end of charge path
      |
      | Create HV On Request block to request charging when vehicle is off
  state HV_Shudown
    state DCDCOFF_Delay
    state Open_Contactors
      entry: MO_BMS_Sollmodus=0;
      HV_State=-1;
      ISO_Hybrid_01_Req = 0;
    state ShutDown_T30C
      entry: T_30C=0;
    state Discharge_Bus
      entry: HVDischarge=1;
      HV_State=-2;
    state Disable_BCM_1
      entry: T_15=0;
      HVDischarge=0;
      HV_State=-3;
    state Disable_BCM_2
      entry: T_30=0;
      HVDischarge=0;
      HV_State=-4;
    state Send_BCM_to_Sleep
      en: MO_SleepAckn =1;
      T_15=0;
      T_30=0;
      HV_State=-5;
    state Shutdown_Complete
      entry: Shutdown_Complete=1;
      HV_State=-6;
    (default) -> DCDCOFF_Delay
    DCDCOFF_Delay -> Open_Contactors : [DCDC_State == 1]
    Open_Contactors -> ShutDown_T30C : after(2,sec)
    ShutDown_T30C -> Discharge_Bus : [BMS_IstModus==5]
    Discharge_Bus -> Disable_BCM_1 : [BMS_Spannung_ZwKr<30]
    Disable_BCM_1 -> Disable_BCM_2 : [BMS_IstStrom<0.02]
    Disable_BCM_2 -> Send_BCM_to_Sleep
    Send_BCM_to_Sleep -> Shutdown_Complete : [BMS_SleepInd]
  note: //Rev 8_21_2017
      | //Removed all engine related conditions
      | //Removed EngRunATV
  note: Need to add a state into Shutdown to wait for all the HV components to be off
      | before opening contactors
  Voltage_Fault -> HV_Shudown [order 1] : after(0.5, sec)
  Ground_Fault -> Fault_light_OFF : [(ISOfault==0&&KeyPos==1)||(ISOfault==0&&KeyPos==0&&plugged==1)]
  HV_Shudown -> Ground_Fault [order 2] : [ISOfault==1]
  Fault_light_OFF -> HV_Shudown
  HV_Startup -> Ground_Fault [order 3] : [ISOfault==1]
  HV_Startup -> HVIL_Fault [order 4] : [BMS_Fehler_Pilot]
  HVIL_Fault -> HV_Shudown : [BMS_Fehler_Pilot==0]
  HV_Startup -> Voltage_Fault [order 1] : after(5,sec)
      | [BMS_Spannung_ZwKr<50&&EngRunAtv]
  Voltage_Fault -> HV_Startup [order 2] : after(1,sec)
  (default) -> HV_Shudown
  HV_Shudown -> HV_Startup [order 1] : [HV_req==1||plugged||EngRunAtv]
  HV_Startup -> HV_Shudown [order 2] : [HV_req==0 && plugged==0]
      | {ReadyToDrive = 0;
      | ReadyToCharge = 0;}
  data: data local; ISOfault input; plugged input; BMS_Fehler_HS_offen input; BMS_Fehler_Pilot input; BMS_Init_abgeschlossen input; BMS_IstModus input; BMS_IstSpannung input; BMS_IstStrom input; BMS_SleepInd input; Diag_Rq_Fktnl_Data_OBD_byte_0 output; Diag_Rq_Fktnl_Data_OBD_byte_1 output; Diag_Rq_Fktnl_Data_OBD_byte_2 output; Diag_Rq_Fktnl_Data_OBD_byte_3 output; Diag_Rq_Fktnl_Data_OBD_byte_4 output; Diag_Rq_Fktnl_Data_OBD_byte_5 output; Diag_Rq_Fktnl_Data_OBD_byte_6 output; Diag_Rq_Fktnl_Data_OBD_byte_7 output; ISO_Hybrid_01_Req output; MO_SleepAckn output; MO_BMS_Sollmodus output; T_15 output; T_30 output; T_30C output; veh_wake output; chga_wake output; HVDischarge output; HV_State output; ReadyToDrive output; ReadyToCharge output; Shutdown_Complete output; HV_req input boolean; BMS_Spannung_ZwKr input; NMH_BMS_Car_WakeUp input; NMH_Normal_Mode_1 input; NMH_BMS_Normal_Mode_2 input; NMH_BMS_Start_1 input; NMH_BMS_Start_2 input; timer local; KeyPos input; GFD_Light output; EngRunAtv input; closeMaincReq input boolean; INV_State input; DCDC_State input

== stateflow chart lib_HVManager_PostIMG_2017a/HV Manager/Invrter Manager/MCU_Manager  ==
  state MCU_Initialization
    state MCU_Request_Standby
      en:
      MCU_State = 1;
      RequestedStateINV = 3;
      CAN_Activation = 1;
    state Power_Off_INVCON
      entry:
      MCU_State = 0;
      INVCON_Power =0;
    state Power_On_INVCON
      en:MCU_State = 2;
      INVCON_Power =1;
    state HV_CAN_Actuation_Fault
      en:
      MCU_State = -1;
      CAN_Activation = 0;
    state INVCON_Power_Fault
      en:
      MCU_State = -2;
      INVCON_Power =0;
      CAN_Activation = 0;
    Power_Off_INVCON -> (junction 18) : {Timer=0;}
    (junction 18) -> MCU_Request_Standby [order 1] : [HVCAN_State]
    (default) -> Power_Off_INVCON
    HV_CAN_Actuation_Fault -> (junction 18) : [HVCAN_State]
    (junction 18) -> HV_CAN_Actuation_Fault [order 2] : after(3,sec)
    INVCON_Power_Fault -> (junction 18) : [~INVCON_Power_Feedback]
    MCU_Request_Standby -> Power_On_INVCON : [HV_State == 9]
    Power_On_INVCON -> INVCON_Power_Fault : after(3,sec)
        | [INV_State ~= 3]
  state MCU_ChargeMode
    state MCU_Ready
      en:
      MCU_State = 7;
    state MCU_Off
      en:
      MCU_State = 8;
      RequestedStateINV = 3;
    (default) -> MCU_ChargeMode.MCU_Ready
    MCU_ChargeMode.MCU_Ready -> MCU_ChargeMode.MCU_Off : [~ReadyToCharge]
  state MCU_TorqueMode
    state MCU_Enable
      en:MCU_State = 4;
      RequestedStateINV = 8;
      during: Timer = Timer + 1;
    state MCU_Ready
      en:
      MCU_State = 3;
    state MCU_Running
      en:
      MCU_State =5;
    state TorqueCommand_Reject_Fault
      en:
      MCU_State = -3;
      RequestedStateINV = 3;
    state MCU_Stop
      en:
      MCU_State = 6;
      RequestedStateINV = 3;
    (default) -> MCU_TorqueMode.MCU_Ready
    MCU_Enable -> (junction 35)
    (junction 35) -> MCU_Running [order 1] : [INV_State == 8]
    MCU_TorqueMode.MCU_Ready -> MCU_Enable : [EnableInverter]
        | {Timer = 0;}
    (junction 35) -> TorqueCommand_Reject_Fault [order 2] : after(10,sec)
    MCU_Running -> MCU_Stop : [~ReadyToDrive]
  state MCU_Shutdown
    state MCU_Off
      en:
      MCU_State = 11;
      RequestedStateINV = 3;
      INVCON_Power = 0;
      Motor_Torque_Command = 0;
    state MCU_Dschrg
      en:
      MCU_State = 10;
      RequestedStateINV = 14;
    state MCU_RdyForShtDwn
      en:
      MCU_State = 9;
    (default) -> MCU_RdyForShtDwn
    MCU_RdyForShtDwn -> MCU_Dschrg : [~EnableInverter]
        | {Timer = 0;}
    MCU_Dschrg -> MCU_Shutdown.MCU_Off : [INV_State == 14 && LinkVoltage<60]
  (default) -> MCU_Initialization
  MCU_Shutdown -> MCU_Initialization : [KeyPos>= 1]
  MCU_TorqueMode -> MCU_Initialization [order 1] : [INV_State == 14]
  MCU_Initialization -> MCU_TorqueMode [order 2] : [INV_State == 3 && INVCON_Power_Feedback && ReadyToDrive]
  MCU_Initialization -> MCU_ChargeMode [order 1] : [INV_State == 3 && INVCON_Power_Feedback && ReadyToCharge]
  MCU_ChargeMode -> MCU_Initialization [order 2] : [INV_State == 14]
  MCU_TorqueMode -> MCU_Shutdown [order 2] : [INV_State == 3 && ~ReadyToDrive]
  MCU_ChargeMode -> MCU_Shutdown [order 1] : [INV_State == 3 && ~ReadyToCharge]
  data: ReadyToDrive input boolean; ReadyToCharge input; HV_State input; HVCAN_State input boolean; INVCON_Power_Feedback input; KeyPos input; LinkVoltage input; INV_State input; INV_CurrentHV input; Timer local double; MCU_State output; EnableInverter input boolean; ShutdownCurrent input; Motor_Torque_Command output; INVCON_Power output double; RequestedStateINV output; CAN_Activation output
